simulink model "ff_controlWeldingRobot"  (R2017b)
settings: Solver=ode23t  StartTime=0.0  StopTime=37  RelTol=1e-3  EnableMultiTasking=on
undefined symbols (not defined in the file or in its folder): p560
libraries: roblocks x5, simulink x2
settings Model: Creator=corkep  LastModifiedBy=ArsalanBangash
settings DataIOCC: LimitDataPoints=on  SaveFormat=Array  SignalLoggingSaveFormat=ModelDataLogs  ReturnWorkspaceOutputs=on  TimeSaveName=t  OutputSaveName=y  ReturnWorkspaceOutputsName=fforward
settings OptimizationCC: ExpressionDepthLimit=2147483647  LifeSpan=inf
settings DebuggingCC: UnderspecifiedInitializationDetection=Classic  MergeDetectMultiDrivingBlocksExec=none  SolverPrmCheckMsg=warning  FcnCallInpInsideContextMsg=warning  AllowSymbolicDim=off  StateNameClashWarn=warning  SFUnexpectedBacktrackingDiag=warning  SFNoUnconditionalDefaultTransitionDiag=warning  SFExecutionAtInitializationDiag=none
settings HardwareCC: ProdBitPerPointer=32  ProdBitPerSizeT=32  ProdBitPerPtrDiffT=32  ProdLargestAtomicFloat=None  ProdIntDivRoundTo=Undefined  ProdEndianess=Unspecified  ProdWordSize=32  ProdHWDeviceType=32-bit Generic
settings ModelReferenceCC: PropagateSignalLabelsOutOfModel=off
settings CodeAppCC: StateflowObjectComments=on
settings GRTTargetCC: TargetLangStandard=C89/C90 (ANSI)  GeneratePreprocessorConditionals=Disable all  CombineOutputUpdateFcns=off  GRTInterface=on
settings ConfigComp: CovMetricSettings=dw  CovHtmlReporting=on  CovSaveCumulativeToWorkspaceVar=on  CovSaveSingleToWorkspaceVar=on  CovExternalEMLEnable=off

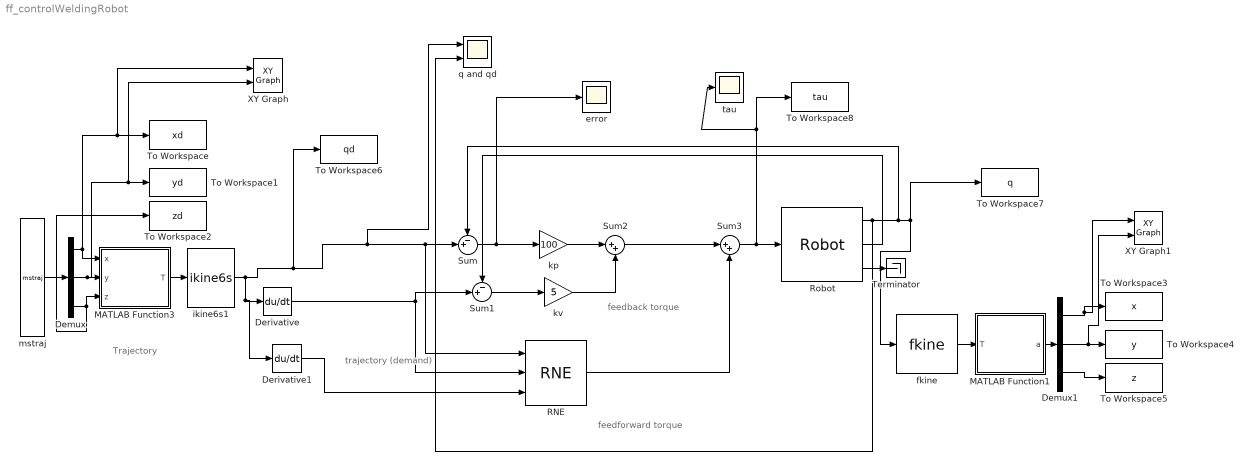
== system ff_controlWeldingRobot ==
  note: feedback torque
  note: trajectory
      | (demand)
  note: feedforward torque
  note: Trajectory
  Demux : Demux  Outputs=3
  Demux1 : Demux  Outputs=3
  Derivative : Derivative
  Derivative1 : Derivative
  MATLAB Function1 : MATLAB Function  TreatAsAtomicUnit=on
  MATLAB Function3 : MATLAB Function  TreatAsAtomicUnit=on
  RNE : roblocks/Arm/RNE  robot=p560.nofriction()  grav=[0 0 9.81]
  Robot : roblocks/Arm/Robot  robot=p560.nofriction  q0=[0 0 0 0 0 0]
  Sum : Sum  Inputs=-+|  SaturateOnIntegerOverflow=on  InputSameDT=on  OutDataTypeStr=Inherit: Same as first input
  Sum1 : Sum  Inputs=-+|  SaturateOnIntegerOverflow=on  InputSameDT=on  OutDataTypeStr=Inherit: Same as first input
  Sum2 : Sum  Inputs=|++  SaturateOnIntegerOverflow=on  InputSameDT=on  OutDataTypeStr=Inherit: Same as first input
  Sum3 : Sum  Inputs=|++  SaturateOnIntegerOverflow=on  InputSameDT=on  OutDataTypeStr=Inherit: Same as first input
  Terminator : Terminator
  To Workspace : ToWorkspace  VariableName=xd  SampleTime=-1
  To Workspace1 : ToWorkspace  VariableName=yd  SampleTime=-1
  To Workspace2 : ToWorkspace  VariableName=zd  SampleTime=-1
  To Workspace3 : ToWorkspace  VariableName=x  SampleTime=-1
  To Workspace4 : ToWorkspace  VariableName=y  SampleTime=-1
  To Workspace5 : ToWorkspace  VariableName=z  SampleTime=-1
  To Workspace6 : ToWorkspace  VariableName=qd  SampleTime=-1
  To Workspace7 : ToWorkspace  VariableName=q  SampleTime=-1
  To Workspace8 : ToWorkspace  VariableName=tau  SampleTime=-1
  XY Graph : simulink/Sinks/XY Graph  xmin=-1  xmax=1  ymin=-1  ymax=1  st=-1
  XY Graph1 : simulink/Sinks/XY Graph  xmin=-1  xmax=1  ymin=-1  ymax=1  st=-1
  error : Scope
  fkine : roblocks/Arm/fkine  robot=p560
  ikine6s1 : roblocks/Arm/ikine6s  robot=p560  conf='luf'
  "kp " : Gain  Gain=100
  "kv " : Gain  Gain=5
  mstraj : roblocks/Toolbox/mstraj  path=|  vaxis=[0.1 0.1 0.1]  tseg=[]  dt=0.1  tacc=0  setsimtime=on
      | [ 0.5,-0.5,0.1;
      |  0.5,-0.5,0.5 ;0.5,0.5,0.5;0.5,0.5,0.1; 0.5,-0.5,0.1; 0.5,-0.5,0.5; 0.5 0 0]
  q and qd : Scope  NumInputPorts=2
  tau : Scope
  wires:
  "kv "/1 -> Sum2/2
  Sum/1 -> "kp "/1, error/1
  "kp "/1 -> Sum2/1
  Sum1/1 -> "kv "/1
  Robot/1 -> q and qd/2, Sum/1, To Workspace7/1, fkine/1
  Robot/2 -> Sum1/1
  ikine6s1/1 -> Derivative1/1, Derivative/1, To Workspace6/1, q and qd/1, RNE/1, Sum/2
  Derivative/1 -> Sum1/2, RNE/2
  Derivative1/1 -> RNE/3
  Robot/3 -> Terminator/1
  RNE/1 -> Sum3/2
  Sum2/1 -> Sum3/1
  MATLAB Function3/1(T) -> ikine6s1/1
  mstraj/1 -> Demux/1
  Demux/2 -> XY Graph/2, To Workspace1/1, MATLAB Function3/2(y)
  Demux/1 -> MATLAB Function3/1(x), XY Graph/1, To Workspace/1
  Demux/3 -> MATLAB Function3/3(z), To Workspace2/1
  fkine/1 -> MATLAB Function1/1(T)
  MATLAB Function1/1(a) -> Demux1/1
  Demux1/1 -> XY Graph1/1, To Workspace3/1
  Demux1/2 -> XY Graph1/2, To Workspace4/1
  Demux1/3 -> To Workspace5/1
  Sum3/1 -> tau/1, To Workspace8/1, Robot/1

== matlab function ff_controlWeldingRobot/MATLAB Function1 ==
  data: T input; a output
function  a= fcn(T)

a=transl(T);

== matlab function ff_controlWeldingRobot/MATLAB Function3 ==
  data: x input; T output; y input; z input
function T = fcn(x,y,z)

T=transl(x,y,z);
